simulink model "Task1_2_Adaptive_Estimator"  (R2024b)
settings: Solver=ode45  StartTime=0.0  StopTime=30  MaxStep=0.01  RelTol=1e-3
InitFcn:
  | if ~exist('params','var'), params=System_Parameters(); end; if ~exist('simcfg','var'), simcfg=Simulink_Config(params); end;
undefined symbols (not defined in the file): params, simcfg
settings Model: Creator=LAPTOPASADI  LastModifiedBy=LAPTOPASADI

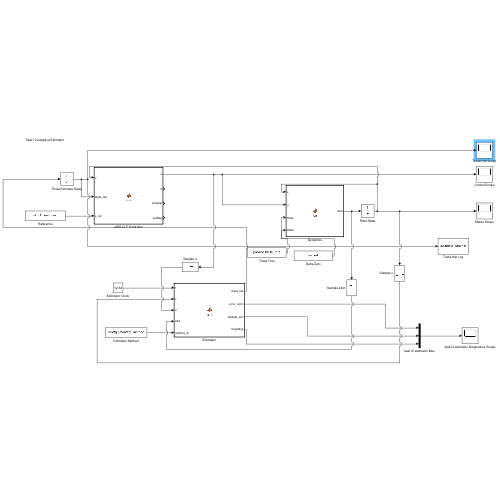
[thumbnail: Simulink's stored preview of the top-level diagram]
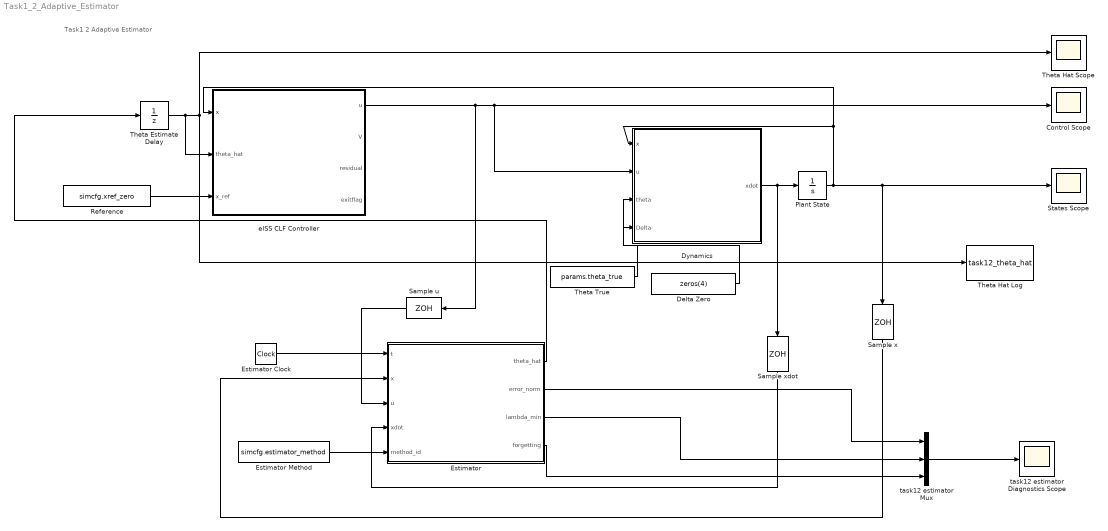
== system Task1_2_Adaptive_Estimator ==
  note: Task1 2 Adaptive Estimator
  Control Scope : Scope
  Delta Zero : Constant  Value=zeros(4)
  Dynamics : MATLAB Function  TreatAsAtomicUnit=on
  Estimator : MATLAB Function  TreatAsAtomicUnit=on
  Estimator Clock : DigitalClock  SampleTime=params.estimator_dt
  Estimator Method : Constant  Value=simcfg.estimator_method
  Plant State : Integrator  InitialCondition=simcfg.x0_task11
  Reference : Constant  Value=simcfg.xref_zero
  Sample u : ZeroOrderHold  SampleTime=params.estimator_dt
  Sample x : ZeroOrderHold  SampleTime=params.estimator_dt
  Sample xdot : ZeroOrderHold  SampleTime=params.estimator_dt
  States Scope : Scope
  Theta Estimate Delay : UnitDelay  InitialCondition=params.theta_hat0  SampleTime=params.estimator_dt  HasFrameUpgradeWarning=on
  Theta Hat Log : ToWorkspace  VariableName=task12_theta_hat  SaveFormat=Structure With Time  SampleTime=-1
  Theta Hat Scope : Scope
  Theta True : Constant  Value=params.theta_true
  eISS CLF Controller : MATLAB Function  TreatAsAtomicUnit=on
  task12 estimator Diagnostics Scope : Scope
  task12 estimator Mux : Mux  Inputs=3
  wires:
  Plant State/1 -> Sample x/1, States Scope/1, eISS CLF Controller/1(x), Dynamics/1(x)
  Theta Estimate Delay/1 -> Theta Hat Scope/1, Theta Hat Log/1, eISS CLF Controller/2(theta_hat)
  Reference/1 -> eISS CLF Controller/3(x_ref)
  eISS CLF Controller/1(u) -> Control Scope/1, Dynamics/2(u), Sample u/1
  Theta True/1 -> Dynamics/3(theta)
  Delta Zero/1 -> Dynamics/4(Delta)
  Dynamics/1(xdot) -> Plant State/1, Sample xdot/1
  Estimator Clock/1 -> Estimator/1(t)
  Sample x/1 -> Estimator/2(x)
  Sample u/1 -> Estimator/3(u)
  Sample xdot/1 -> Estimator/4(xdot)
  Estimator Method/1 -> Estimator/5(method_id)
  Estimator/1(theta_hat) -> Theta Estimate Delay/1
  Estimator/2(error_norm) -> task12 estimator Mux/1
  Estimator/3(lambda_min) -> task12 estimator Mux/2
  Estimator/4(forgetting) -> task12 estimator Mux/3
  task12 estimator Mux/1 -> task12 estimator Diagnostics Scope/1

== matlab function Task1_2_Adaptive_Estimator/Dynamics ==
  data: x input; u input; xdot output; theta input; Delta input
function xdot = fcn(x,u,theta,Delta)
G = [0 0 40.75371832714017 8.6858779355964231;0 5.9859154929577469 0 0;0 0 2.4098880670272087 -9.893830239002293];
x=reshape(x,6,1);
u=reshape(u,4,1);
theta=reshape(theta,6,1);
Delta=reshape(Delta,4,4);

phi = x(1);
pitch = x(2);
p = x(4);
q = x(5);
r = x(6);

cphi = cos(phi);
sphi = sin(phi);
cpitch = cos(pitch);
if abs(cpitch) < 1e-6
    cpitch = sign(cpitch+eps)*1e-6;
end
tpitch = sin(pitch)/cpitch;

J = [1, sphi*tpitch, cphi*tpitch;
     0, cphi,         -sphi;
     0, sphi/cpitch,  cphi/cpitch];
f0 = [J*[p;q;r]; zeros(3,1)];
Fomega = [p*q, -q*r, 0, 0, 0, -p;
          0, 0, p*r, -(p^2-r^2), 0, -q;
          -q*r, 0, 0, 0, p*q, -r];
F = [zeros(3,6); Fomega];
g = [zeros(3,4); G];
xdot = f0+F*theta+g*(eye(4)+Delta)*u;
end

== matlab function Task1_2_Adaptive_Estimator/eISS CLF Controller ==
  data: x input; u output; theta_hat input; x_ref input; V output; residual output; exitflag output
function [u,V,residual,exitflag] = fcn(x,theta_hat,x_ref)
P = [0.11250000000000002 0 0 0.012500000000000001 0 0;0 0.11250000000000002 0 0 0.012500000000000001 0;0 0 0.11250000000000002 0 0 0.012500000000000001;0.012500000000000001 0 0 0.015625 0 0;0 0.012500000000000001 0 0 0.015625 0;0 0 0.012500000000000001 0 0 0.015625];
G = [0 0 40.75371832714017 8.6858779355964231;0 5.9859154929577469 0 0;0 0 2.4098880670272087 -9.893830239002293];
x=reshape(x,6,1);
theta_hat=reshape(theta_hat,6,1);
x_ref=reshape(x_ref,6,1);
c_eiss = 0.5;
kappa = 10;
lower = [-0.10000000000000001;-0.10000000000000001;-0.10000000000000001;-0.10000000000000001];
upper = [0.10000000000000001;0.10000000000000001;0.10000000000000001;0.10000000000000001];

[V,omega,phiV,LgV] = clf_terms(x,x_ref,P,G);
iota = (phiV'*phiV)/kappa;
b = -c_eiss*V+iota-omega-phiV'*theta_hat;
[u,exitflag] = project_origin(LgV,b,lower,upper);
residual = omega+phiV'*theta_hat+LgV*u+c_eiss*V-iota;
end

function [V,omega,phiV,LgV] = clf_terms(x,x_ref,P,G)
phi = x(1); pitch = x(2); w = x(4:6);
[J,Jphi,Jpitch] = kinematics(phi,pitch);
rates = J*w;
Jdot = Jphi*rates(1)+Jpitch*rates(2);
eta = [x(1:3)-x_ref(1:3); rates];
p = x(4); q = x(5); r = x(6);
Fw = [p*q,-q*r,0,0,0,-p; 0,0,p*r,-(p^2-r^2),0,-q; -q*r,0,0,0,p*q,-r];
grad = 2*P*eta;
V = eta'*P*eta;
omega = grad(1:3)'*rates+grad(4:6)'*(Jdot*w);
phiV = (J*Fw)'*grad(4:6);
LgV = grad(4:6)'*(J*G);
end

function [J,Jphi,Jpitch] = kinematics(phi,pitch)
c = cos(phi); s = sin(phi); cp = cos(pitch);
if abs(cp)<1e-6, cp=sign(cp+eps)*1e-6; end
t = sin(pitch)/cp; sec = 1/cp;
J = [1,s*t,c*t; 0,c,-s; 0,s*sec,c*sec];
Jphi = [0,c*t,-s*t; 0,-s,-c; 0,c*sec,-s*sec];
Jpitch = [0,s*sec^2,c*sec^2; 0,0,0; 0,s*sec*t,c*sec*t];
end

function [u,flag] = project_origin(a,b,lower,upper)
tol = 1e-12;
u = min(max(zeros(4,1),lower),upper);
if a*u <= b+tol, flag=1; return; end
umin = upper; umin(a>=0)=lower(a>=0);
if a*umin > b+tol, u=umin; flag=-2; return; end
lo=0; hi=1;
while a*min(max(-hi*a',lower),upper) > b
    hi=2*hi;
    if hi>1e12, u=umin; flag=-2; return; end
end
for k=1:80
    mid=0.5*(lo+hi); candidate=min(max(-mid*a',lower),upper);
    if a*candidate>b, lo=mid; else, hi=mid; end
end
u=min(max(-hi*a',lower),upper); flag=1;
end

== matlab function Task1_2_Adaptive_Estimator/Estimator ==
  data: t input; x input; u input; theta_hat output; xdot input; method_id input; error_norm output; lambda_min output; forgetting output
function [theta_hat,error_norm,lambda_min,forgetting] = fcn(t,x,u,xdot,method_id)
persistent theta Pcov Lstack Ystack H b count replay last_t last_method last_lambda

N = 20;
dt = 0.01;
theta0 = [0;0.5;0.5;0;-0.29999999999999999;0];
G = [0 0 40.75371832714017 8.6858779355964231;0 5.9859154929577469 0 0;0 0 2.4098880670272087 -9.893830239002293];
x=reshape(x,6,1);
u=reshape(u,4,1);
xdot=reshape(xdot,6,1);

method_now = min(4,max(1,round(method_id)));
if isempty(theta), theta=theta0; end
if isempty(Pcov), Pcov=100*eye(6); end
if isempty(Lstack), Lstack=zeros(6,6,N); end
if isempty(Ystack), Ystack=zeros(6,N); end
if isempty(H), H=zeros(6); end
if isempty(b), b=zeros(6,1); end
if isempty(count), count=0; end
if isempty(replay), replay=1; end
if isempty(last_t), last_t=-inf; end
if isempty(last_method), last_method=method_now; end
if isempty(last_lambda), last_lambda=1; end

reset = (t < last_t-0.5*dt) || (method_now ~= last_method);
if reset
    theta=theta0;
    Pcov=100*eye(6);
    Lstack=zeros(6,6,N);
    Ystack=zeros(6,N);
    H=zeros(6);
    b=zeros(6,1);
    count=0;
    replay=1;
    last_t=-inf;
    last_method=method_now;
    last_lambda=1;
end

p=x(4); q=x(5); r=x(6);
L=[zeros(3,6); p*q,-q*r,0,0,0,-p; 0,0,p*r,-(p^2-r^2),0,-q; -q*r,0,0,0,p*q,-r];
[f0,g] = nominal_terms(x,G);
Y = xdot-f0-g*u;
if 0 > 0
    Y = Y+0*randn(6,1);
end
error_norm = norm(Y-L*theta);

if t > last_t+0.25*dt
    [Lstack,Ystack,H,b,count,lambda_min] = update_stack( ...
        Lstack,Ystack,H,b,count,L,Y,N);
    method = method_now;
    if method==1
        e=Y-L*theta;
        theta_dot=[10 0 0 0 0 0;0 10 0 0 0 0;0 0 10 0 0 0;0 0 0 10 0 0;0 0 0 0 10 0;0 0 0 0 0 10]*(L'*e+5*(b-H*theta));
        theta=theta+dt*theta_dot;
        forgetting=1;
    else
        forgetting=1;
        if method==3
            forgetting=0.995;
        elseif method==4
            e=Y-L*theta;
            normalized=(e'*e)/(1e-08+Y'*Y);
            rho=20*normalized;
            forgetting=1-(1-0.96999999999999997)*rho/(1+rho);
            if norm(L,'fro')<0.0001
                forgetting=1;
            end
            forgetting=min(1,max(0.96999999999999997,forgetting));
        end
        [theta,Pcov]=rls_step(theta,Pcov,L,Y,forgetting, ...
            1e-08,100000);
        if count>0
            index=min(replay,count);
            [theta,Pcov]=rls_step(theta,Pcov,Lstack(:,:,index), ...
                Ystack(:,index),1,1e-08,100000);
            replay=mod(index,count)+1;
        end
        if method==4
            Pcov=clip_cov(Pcov,9.9999999999999995e-07,1000);
        end
    end
    last_lambda=forgetting;
    last_t=t;
else
    forgetting=last_lambda;
    lambda_min=min_eig(H);
end
theta_hat=theta;
end

function [f0,g]=nominal_terms(x,G)
phi=x(1); pitch=x(2); w=x(4:6);
c=cos(phi); s=sin(phi); cp=cos(pitch);
if abs(cp)<1e-6, cp=sign(cp+eps)*1e-6; end
t=sin(pitch)/cp;
J=[1,s*t,c*t;0,c,-s;0,s/cp,c/cp];
f0=[J*w;zeros(3,1)];
g=[zeros(3,4);G];
end

function [Ls,Ys,H,b,count,lambda_min]=update_stack(Ls,Ys,H,b,count,L,Y,N)
if norm(L,'fro')<1.0000000000000001e-05
    lambda_min=min_eig(H); return;
end
if count<N
    count=count+1; Ls(:,:,count)=L; Ys(:,count)=Y;
    H=H+L'*L; b=b+L'*Y;
else
    current=min_eig(H); best=current; best_index=0; bestH=H;
    for index=1:N
        old=Ls(:,:,index);
        candidate=H-old'*old+L'*L;
        value=min_eig(candidate);
        if value>best+1e-10
            best=value; best_index=index; bestH=candidate;
        end
    end
    if best_index>0
        old=Ls(:,:,best_index); oldY=Ys(:,best_index);
        Ls(:,:,best_index)=L; Ys(:,best_index)=Y;
        H=bestH; b=b-old'*oldY+L'*Y;
    end
end
lambda_min=min_eig(H);
end

function value=min_eig(A)
value=max(0,min(real(eig(0.5*(A+A')))));
end

function [theta,P]=rls_step(theta,P,L,Y,lambda,lower,upper)
S=lambda*eye(6)+L*P*L';
K=(P*L')/S;
theta=theta+K*(Y-L*theta);
P=(P-K*L*P)/lambda;
P=clip_cov(P,lower,upper);
end

function P=clip_cov(P,lower,upper)
[vectors,values]=eig(0.5*(P+P'));
vectors=real(vectors);
d=min(max(real(diag(values)),lower),upper);
P=vectors*diag(d)*vectors';
P=0.5*(P+P');
end
